simulink model "FYPrefer"  (R2025b)
settings: Solver=ode23  StartTime=0.0  StopTime=1  MaxStep=1e-3  RelTol=1e-4  AbsTol=1e-6
libraries: ee_lib x32, fl_lib x21, nesl_utility x5, simulink x1
settings Model: Creator=30807  LastModifiedBy=30807
settings DebuggingCC: SignalInfNanChecking=warning  SignalRangeChecking=warning  AlgebraicLoopMsg=error  ArtificialAlgebraicLoopMsg=error  BlockPriorityViolationMsg=error  MinStepSizeMsg=error  TimeAdjustmentMsg=warning  SolverPrmCheckMsg=warning  SingleTaskRateTransMsg=warning  CheckMatrixSingularityMsg=warning  ParameterUnderflowMsg=warning  UnderSpecifiedDataTypeMsg=warning  UnnecessaryDatatypeConvMsg=warning  VectorMatrixConversionMsg=warning  SignalLabelMismatchMsg=warning  UnconnectedInputMsg=warning  UnconnectedOutputMsg=warning  UnconnectedLineMsg=warning  SFcnCompatibilityMsg=warning  ModelReferenceVersionMismatchMessage=warning  ModelReferenceIOMismatchMessage=warning  ModelReferenceNoExplicitFinalValueMsg=warning  StateNameClashWarn=warning  StrictBusMsg=WarnOnBusTreatedAsVector  NonBusSignalsTreatedAsBus=warning  UnderSpecifiedDimensionMsg=warning

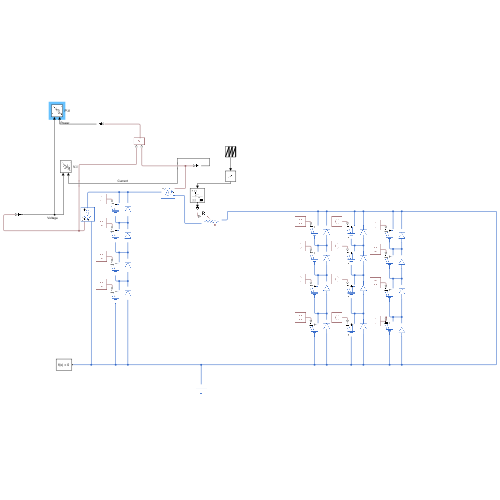
[thumbnail: Simulink's stored preview of the top-level diagram]
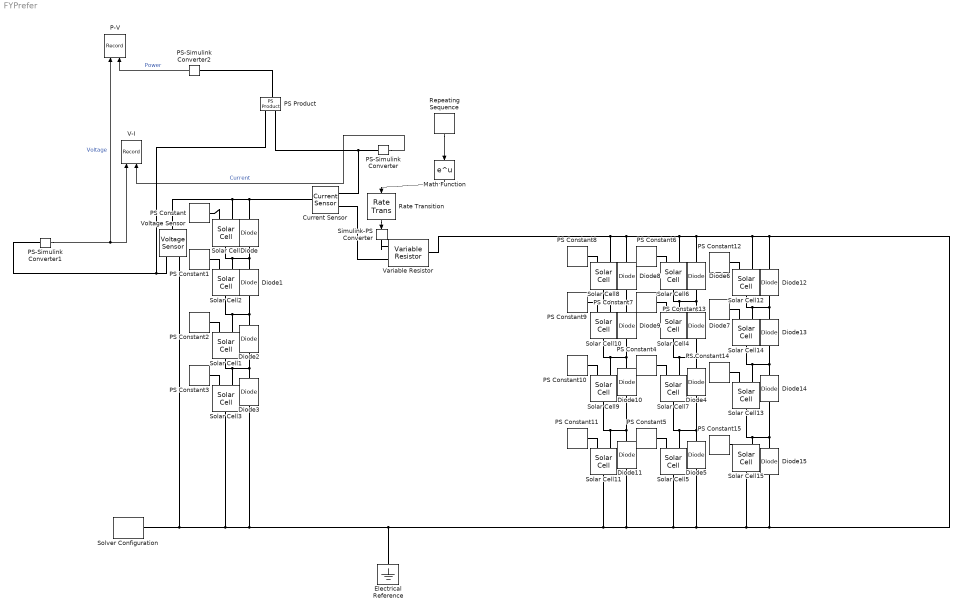
== system FYPrefer ==
  Current Sensor : fl_lib/Electrical/Electrical Sensors/Current Sensor
  Diode{,1..15} (16 alike) : ee_lib/Semiconductors & Converters/Diode  ModelType=ee.enum.diode.modelType.pwl  TableType=ee.enum.diode.tableType.IfMat  IfMat=[.07, .12, .19, 1.75, 4.24, 7.32, 11.2; .16, .3, .72, 2.14, 5.02, 8.35, 13.12] A  VfMat=[.9, 1.15, 1.25, 1.5, 1.75, 2.17, 2.6, 2.85; .58, .68, .75, 1.1, 1.38, 1.77, 2.27, 2.7] V  TjVec=[25, 125] degC  VfVec=[.5, .7, .9, 1.3, 1.7, 2.1, 2.5] V  IfVec=[.1, .2, .5, 1, 2, 4, 7, 10] A  IrMat=[1e-06, 2e-06, 5e-06, 1e-05, 2.5e-05, 5e-05, .0001; 2e-06, 5e-06, 1e-05, 4e-05, 8e-05, .0002, .0005] A  VrMat=[10, 100, 200, 250, 300, 325, 350; 10, 70, 160, 220, 270, 300, 320] V  VrVec=[10, 20, 40, 50, 70, 80, 100] V  IrVec=[1e-06, 2e-06, 5e-06, 1e-05, 2e-05, 5e-05, .0001] A  Vf=0.6 V  Ron=1e-2 Ohm  Goff=1e-8 S  prmExp=ee.enum.diode.expParam.useTwo  I12=[.0137, .545] A  V12=[.6, .7] V  RS=0 Ohm  Tmeas=298.15 K  IS=1e-12 A  ec=1  I1=0.0137 A  V1=0.6 V  N_series=1  N_parallel=1  ZenerEnable=false  Rz=0.3 Ohm  BV=inf V  C_param=ee.enum.diode.capParam.fixed  CJ=0 pF  CJ0=5 pF  Vvec=[.1, 10, 100] V  Cvec=[3.5, 1, .4] pF  VJ=1 V  Mgrad=0.5  FC=0.5  Q_param=ee.enum.diode.recoveryParam.off  iRM=-7.15 A  iF=4 A  didt=-750 A/us  trr_factor=3  trr=115 ns  Qrr=150 nA*s  Vr=-600 V  Ls=150 nH  Erec=0.03 J  TT=50 ns  tau=100 ns  T_param=ee.enum.diode.temperatureParam.off  Tdevice=298.15 K  I1_T2=0.245 A  V1_T2=0.5 V  IS_T2=1.25e-7 A  Tmeas2=125 degC  XTI_param=ee.enum.diode.xtiParam.pn  XTI=3  EG_param=ee.enum.diode.egapParam.material_si  EG=1.11 eV  dBVdT=0 V/K  enable_fault_input=simscape.enum.onoff.off  i_specify=off  i_priority=None  i=0 A  i_nominal_specify=off  i_nominal_value=1  i_nominal_unit=A  v_specify=off  v_priority=None  v=0 V  v_nominal_specify=off  v_nominal_value=1  v_nominal_unit=V  v_capacitor_specify=off  v_capacitor_priority=None  v_capacitor=0 V  v_capacitor_nominal_specify=off  v_capacitor_nominal_value=1  v_capacitor_nominal_unit=V  Qj_specify=off  Qj_priority=High  Qj=0 C  Qj_nominal_specify=off  Qj_nominal_value=1  Qj_nominal_unit=C  i_diode_specify=off  i_diode_priority=None  i_diode=0 A  i_diode_nominal_specify=off  i_diode_nominal_value=1  i_diode_nominal_unit=A  v_diode_specify=off  v_diode_priority=None  v_diode=0 V  v_diode_nominal_specify=off  v_diode_nominal_value=1  v_diode_nominal_unit=V  i_capacitor_specify=off  i_capacitor_priority=None  i_capacitor=0 A  i_capacitor_nominal_specify=off  i_capacitor_nominal_value=1  i_capacitor_nominal_unit=A  power_dissipated_specify=off  power_dissipated_priority=None  power_dissipated=0 W  power_dissipated_nominal_specify=off  power_dissipated_nominal_value=1  power_dissipated_nominal_unit=W  fidelity_level=ee.enum.diode.fidelity.includeChargeDyn  rec_loss_model=ee.enum.diode.reverseRecoveryModel.fixed  ErecVal=0 J  scaleWithIandV=true  ErecMat=zeros(2, 3) J  TjrecVec=[298.15, 398.15] K  IfrecVec=[.1, 1, 10] A  IrecVal=10 A  VrecVal=10 V  tFilter=1 / 1000 / 100 s  thermal_network_parameterization=ee.enum.thermalNetworkTopology.junctionCase  Rth=[0, 10] K/W  Rth_Cauer=[1, 3, 10] K/W  Rth_Foster=[.08, .14, .22, .16] K/W  thermal_mass_parameterization=ee.enum.thermalNetwork.timeconstant  thermal_mass=[0, 1] J/K  thermal_mass_Cauer=[.1, .3, 1] J/K  thermal_mass_Foster=[.001, .005, .05, .5] J/K  thermal_time_constant=[0, 10] s  thermal_time_constant_Cauer=[1, 3, 10] s  thermal_time_constant_Foster=[7e-05, .0007, .01, .08] s  thermal_mass_initial_temperatures=[25, 25] degC  thermal_mass_initial_temperatures_Cauer=[25, 25, 25] degC  junction_thermal_mass=0.01 J/K  Tvec_initial_Foster=[25, 25, 25, 25] degC  no_thermal_network=0  junction_temperature_specify=off  junction_temperature_priority=None  junction_temperature=25 degC  junction_temperature_nominal_specify=off  junction_temperature_nominal_value=1  junction_temperature_nominal_unit=degC
  Electrical Reference : fl_lib/Electrical/Electrical Elements/Electrical Reference
  Math Function : Math
  P-V : Record  NumPorts=2.0  FileSettingsInternal="{\"entries\":[{\"content\":{\"excelSettings\":{\"content\":{},\"type\":\"Streamout.ExcelSettings\"},\"parquetSettings\":{\"content\":{},\"type\":\"Streamout.ParquetSettings\"}},\"type\":\"Streamout.FileSettingStorage\",\"uuid\":\"\"}],\"packageUris\":[\"http:\\/\\/schema.mathworks.com\\/mf0\\/streamout_blocks\\/R2020a\"],\"version\":\"1.0\"}"  FrameSettings=[0, 0]  Layout=[1 1]  SignalsInternal="{\"entries\":[{\"content\":{\"signals\":[{\"content\":{\"blockPath\":[],\"dimensions\":[1],\"domain\":\"\",\"lineColor\":\"#77ac30\",\"lineWidth\":2,\"plots\":[ 1 ],\"port\":1,\"sid\":[\"\"],\"signalID\":1,\"signalName\":\"Voltage\"},\"type\":\"RecordBlkView.Signal\",\"uuid\":\"\"},{\"content\":{\"blockPath\":[],\"dimensions\":[1],\"domain\":\"\",\"lineColor\":\"#4dbeee\",\"lineWidth\":2,\"plots\":[ 1 ],\"port\":2,\"sid\":[\"\"],\"signalID\":2,\"signalName\":\"Power\"},\"type\":\"RecordBlkView.Signal\",\"uuid\":\"\"}]},\"type\":\"RecordBlkView.InputSignals\",\"uuid\":\"\"}],\"packageUris\":[\"http:\\/\\/schema.mathworks.com\\/mf0\\/streamout_blocks\\/R2020a\"],\"version\":\"1.0\"}"  VisualizationBindings="{\"xyplotplugin\":{\"info\":[{\"series\":[{\"bindingParametersList\":[{\"parameter\":\"X-Axis\",\"signalID\":1,\"signalName\":\"Voltage\"},{\"parameter\":\"Y-Axis\",\"signalID\":2,\"signalName\":\"Power\"}],\"seriesID\":0}],\"subplotID\":1}]}}"  CompatibilityTag=XY
  PS Constant{,1,4..9,12..15} (12 alike) : fl_lib/Physical Signals/Sources/PS Constant  constant=1000 W/m^2
  PS Constant{2..3,10..11} (4 alike) : fl_lib/Physical Signals/Sources/PS Constant  constant=500 W/m^2
  PS Product : fl_lib/Physical Signals/Functions/PS Product
  PS-Simulink Converter : nesl_utility/PS-Simulink Converter  PhysicalDomain=network_engine_domain  SubClassName=ps_output  LeftPortType=input  RightPortType=output  PseudoPeriodic=off  Frequencies=[]  VectorFormat=inherit  Unit=A  AffineConversion=off
  PS-Simulink Converter1 : nesl_utility/PS-Simulink Converter  PhysicalDomain=network_engine_domain  SubClassName=ps_output  LeftPortType=input  RightPortType=output  PseudoPeriodic=off  Frequencies=[]  VectorFormat=inherit  Unit=V  AffineConversion=off
  PS-Simulink Converter2 : nesl_utility/PS-Simulink Converter  PhysicalDomain=network_engine_domain  SubClassName=ps_output  LeftPortType=input  RightPortType=output  PseudoPeriodic=off  Frequencies=[]  VectorFormat=inherit  Unit=W  AffineConversion=off
  Rate Transition : RateTransition  OutPortSampleTime=1e-5
  Repeating Sequence : simulink/Sources/Repeating Sequence  rep_seq_t=[0 1]  rep_seq_y=[-6.9078 13.8155]
  Simulink-PS Converter : nesl_utility/Simulink-PS Converter  PhysicalDomain=network_engine_domain  SubClassName=ps_input  LeftPortType=input  RightPortType=output  PseudoPeriodic=off  Frequencies=[]  NoiseDistribution=none  NoiseParameters=[]  Unit=Ohm  AffineConversion=off  FilteringAndDerivatives=provide  SimscapeFilterOrder=1  InputFilterTimeConstant=0.001  UdotUserProvided=0
  Solar Cell{,6,8,12} (4 alike) : ee_lib/Sources/Solar Cell  prm=ee.enum.sources.solar_cell_prm.fiveParameter  Isc=1.27 % Datasheet derived A  Voc=0.92227 % Datasheet derived V  Is=3.9947e-8 A  Is2=2.18760100392676e-13 % Datasheet derived A  Iph=4.75 A  Ir0=1000 W/m^2  ec=1.2  N2=1.20419611511633 % Datasheet derived  Rs=0.013888 Ohm  Rp=9038.61907734448 % Datasheet derived Ohm  N_series=72  N_parallel=1  TIPH1=0.00065 1/K  EG=1.15 eV  TXIS1=3  TXIS2=3  TRS1=0  TRP1=0  Tmeas=25 degC  TFIXED=25 degC  thermal_mass=100 J/K  initial_temperature=25 degC
  Solar Cell{1..5,7,9..11,13..15} (12 alike) : ee_lib/Sources/Solar Cell  prm=ee.enum.sources.solar_cell_prm.fiveParameter  Isc=4.75 A  Voc=43.5 V  Is=3.9947e-8 A  Is2=0 A  Iph=4.75 A  Ir0=1000 W/m^2  ec=1.2  N2=2  Rs=0.013888 Ohm  Rp=inf Ohm  N_series=72  N_parallel=1  TIPH1=0.00065 1/K  EG=1.15 eV  TXIS1=3  TXIS2=3  TRS1=0  TRP1=0  Tmeas=25 degC  TFIXED=25 degC  thermal_mass=100 J/K  initial_temperature=25 degC
  Solver Configuration : nesl_utility/Solver Configuration  PhysicalDomain=network_engine_domain  SubClassName=solver  LeftPortType=input  RightPortType=generic  Tones=[]  Harmonics=[]  SimulateNoise=off  Profile=off  UseLocalSampling=off  EnableSwitchedLinearOptims=on  FrequencyDomain=off  UseCCode=off  RelTol=0.001  AbsTol=0.001  MinStep=1e-09  ToWorkspace=off  RevertToSquareIcSolve=off  NumHomotopyIterations=100  PhasorMode=off  PhasorModeNumHarmonics=1  ConsistencySolver=NEWTON_XTOL_AFTER_FTOL  IndexReductionMethod=DerivativeReplacement  DoDC=off  ResidualTolerance=1e-09  ConsistencyTolSource=GLOBAL  ConsistencyAbsTol=0.001  ConsistencyRelTol=0.001  ConsistencyTolFactor=0.001  UseLocalSolver=on  LocalSolverChoice=NE_BACKWARD_EULER_ADVANCER  ResolveIndetEquations=off  FunctionEvalNumThread=1  LocalSolverSampleTime=0.00001  DoFixedCost=off  MaxNonlinIter=3  MaxModeIter=2  ComputeImpulses=off  ImpulseIterations=2  LinearAlgebra=auto  LinearAlgebraNumThread=0  EquationFormulation=NE_TIME_EF  DelaysMemoryBudget=1024  AutomaticFiltering=off  FilteringTimeConstant=0.001  PartitionStorageMethod=AS_NEEDED  PartitionMemoryBudget=1024  PartitionMethod=ROBUST  MultibodyUseLocalSolver=off  MultibodyLocalSolverChoice=ODE1  MultibodyLocalSolverSampleTime=0.00001
  V-I : Record  NumPorts=2.0  FileSettingsInternal="{\"entries\":[{\"content\":{\"excelSettings\":{\"content\":{},\"type\":\"Streamout.ExcelSettings\"},\"parquetSettings\":{\"content\":{},\"type\":\"Streamout.ParquetSettings\"}},\"type\":\"Streamout.FileSettingStorage\",\"uuid\":\"\"}],\"packageUris\":[\"http:\\/\\/schema.mathworks.com\\/mf0\\/streamout_blocks\\/R2020a\"],\"version\":\"1.0\"}"  FrameSettings=[0, 0]  Layout=[1 1]  SignalsInternal="{\"entries\":[{\"content\":{\"signals\":[{\"content\":{\"blockPath\":[],\"dimensions\":[1],\"domain\":\"\",\"lineColor\":\"#a2142f\",\"lineWidth\":2,\"plots\":[ 1 ],\"port\":1,\"sid\":[\"\"],\"signalID\":1,\"signalName\":\"Voltage\"},\"type\":\"RecordBlkView.Signal\",\"uuid\":\"\"},{\"content\":{\"blockPath\":[],\"dimensions\":[1],\"domain\":\"\",\"lineColor\":\"#139fff\",\"plots\":[ 1 ],\"port\":2,\"sid\":[\"\"],\"signalID\":2,\"signalName\":\"Current\"},\"type\":\"RecordBlkView.Signal\",\"uuid\":\"\"}]},\"type\":\"RecordBlkView.InputSignals\",\"uuid\":\"\"}],\"packageUris\":[\"http:\\/\\/schema.mathworks.com\\/mf0\\/streamout_blocks\\/R2020a\"],\"version\":\"1.0\"}"  VisualizationBindings="{\"xyplotplugin\":{\"info\":[{\"series\":[{\"bindingParametersList\":[{\"parameter\":\"X-Axis\",\"signalID\":1,\"signalName\":\"Voltage\"},{\"parameter\":\"Y-Axis\",\"signalID\":2,\"signalName\":\"Current\"}],\"seriesID\":0}],\"subplotID\":1}]}}"  CompatibilityTag=XY
  Variable Resistor : fl_lib/Electrical/Electrical Elements/Variable Resistor  Rmin=0.001 Ohm  thermalEnable=false  thermal_mass=1 J/K  i_specify=off  i_priority=None  i=0 A  i_nominal_specify=off  i_nominal_value=1  i_nominal_unit=A  v_specify=off  v_priority=None  v=0 V  v_nominal_specify=off  v_nominal_value=1  v_nominal_unit=V  T_specify=off  T_priority=None  T=300 K  T_nominal_specify=off  T_nominal_value=1  T_nominal_unit=K
  Voltage Sensor : fl_lib/Electrical/Electrical Sensors/Voltage Sensor
  wires:
  Repeating Sequence/1 -> Math Function/1
  Rate Transition/1 -> Simulink-PS Converter/1
  Math Function/1 -> Rate Transition/1
  PS-Simulink Converter2/1 -> P-V/2  "Power"
  PS-Simulink Converter/1 -> V-I/2  "Current"
  PS-Simulink Converter1/1 -> V-I/1, P-V/1  "Voltage"
  connections:
  Solar Cell2/LConn2 -- Diode1/RConn1 -- Diode/LConn1 -- Solar Cell/RConn1
  Current Sensor/LConn1 -- Diode/RConn1 -- Voltage Sensor/LConn1 -- Solar Cell/LConn2
  Electrical Reference/LConn1 -- Diode6/RConn1 -- Diode8/RConn1 -- Solar Cell8/LConn2 -- Variable Resistor/RConn1 -- Solar Cell6/LConn2 -- Solar Cell12/LConn2 -- Diode12/RConn1 -- Diode15/LConn1 -- Solar Cell15/RConn1 -- Diode5/LConn1 -- Solar Cell5/RConn1 -- Diode11/LConn1 -- Solar Cell11/RConn1 -- Diode3/LConn1 -- Solar Cell3/RConn1 -- Voltage Sensor/RConn2 -- Solver Configuration/RConn1
  Current Sensor/RConn2 -- Variable Resistor/LConn2
  Solar Cell/LConn1 -- PS Constant/RConn1
  Solar Cell2/LConn1 -- PS Constant1/RConn1
  Voltage Sensor/RConn1 -- PS Product/LConn1 -- PS-Simulink Converter1/LConn1
  PS-Simulink Converter/LConn1 -- PS Product/LConn2 -- Current Sensor/RConn1
  PS Product/RConn1 -- PS-Simulink Converter2/LConn1
  Simulink-PS Converter/RConn1 -- Variable Resistor/LConn1
  PS Constant2/RConn1 -- Solar Cell1/LConn1
  Solar Cell2/RConn1 -- Diode1/LConn1 -- Diode2/RConn1 -- Solar Cell1/LConn2
  Diode10/RConn1 -- Diode9/LConn1 -- Solar Cell10/RConn1 -- Solar Cell9/LConn2
  Diode11/RConn1 -- Diode10/LConn1 -- Solar Cell9/RConn1 -- Solar Cell11/LConn2
  Diode8/LConn1 -- Solar Cell10/LConn2 -- Solar Cell8/RConn1 -- Diode9/RConn1
  Diode6/LConn1 -- Solar Cell4/LConn2 -- Solar Cell6/RConn1 -- Diode7/RConn1
  Solar Cell7/LConn2 -- Diode7/LConn1 -- Diode4/RConn1 -- Solar Cell4/RConn1
  Diode5/RConn1 -- Diode4/LConn1 -- Solar Cell7/RConn1 -- Solar Cell5/LConn2
  Diode15/RConn1 -- Diode14/LConn1 -- Solar Cell13/RConn1 -- Solar Cell15/LConn2
  Diode12/LConn1 -- Solar Cell14/LConn2 -- Solar Cell12/RConn1 -- Diode13/RConn1
  Diode14/RConn1 -- Diode13/LConn1 -- Solar Cell14/RConn1 -- Solar Cell13/LConn2
  Solar Cell14/LConn1 -- PS Constant13/RConn1
  PS Constant14/RConn1 -- Solar Cell13/LConn1
  PS Constant11/RConn1 -- Solar Cell11/LConn1
  PS Constant12/RConn1 -- Solar Cell12/LConn1
  PS Constant4/RConn1 -- Solar Cell7/LConn1
  Solar Cell10/LConn1 -- PS Constant9/RConn1
  Solar Cell4/LConn1 -- PS Constant7/RConn1
  PS Constant15/RConn1 -- Solar Cell15/LConn1
  PS Constant10/RConn1 -- Solar Cell9/LConn1
  PS Constant5/RConn1 -- Solar Cell5/LConn1
  PS Constant3/RConn1 -- Solar Cell3/LConn1
  Solar Cell3/LConn2 -- Solar Cell1/RConn1 -- Diode2/LConn1 -- Diode3/RConn1
  PS Constant8/RConn1 -- Solar Cell8/LConn1
  PS Constant6/RConn1 -- Solar Cell6/LConn1
